simulink model "TestePlano"  (R2020b)
settings: Solver=FixedStepDiscrete  StartTime=0.0  StopTime=Plano.Tempo(end)  FixedStep=1  RelTol=1e-3
InitFcn:
  |  Plano=readtable('PlanoExperimentos.xlsx');
settings Model: Creator=leize  LastModifiedBy=leize

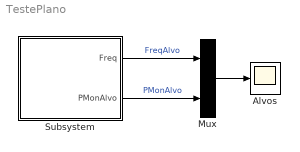
== system TestePlano ==
  Alvos : Scope
  Mux : Mux  Inputs=2
  Subsystem : Subsystem  mask{Plano=Plano}
      mask prompts: Plano "Plano de Execucao"
      mask DialogControl DescGroupVar Prompt: TABELA COM PLANO DE EXECUCAO
  wires:
  Mux/1 -> Alvos/1
  Subsystem/1(Freq) -> Mux/1  "FreqAlvo"
  Subsystem/2(PMonAlvo) -> Mux/2  "PMonAlvo"

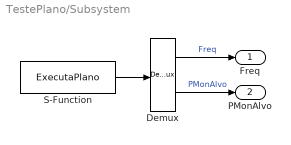
== system TestePlano/Subsystem ==
  Demux : Demux  Outputs=2
  S-Function : S-Function  FunctionName=ExecutaPlano  Parameters=Plano  SFunctionDeploymentMode=off  EnableBusSupport=off
  Freq : Outport
  PMonAlvo : Outport  Port=2
  wires:
  S-Function/1 -> Demux/1
  Demux/1 -> Freq/1  "Freq"
  Demux/2 -> PMonAlvo/1  "PMonAlvo"
